simulink model "sim_adc_2nd_1bit_combfilterfix"  (R2022a)
settings: Solver=FixedStepDiscrete  StartTime=0.0  StopTime=Tstop  RelTol=1e-3  EnableMultiTasking=on
values from neighbouring files (symbols this model uses):
  a1 = 0.7752    [Sigmadelta_1bit_CIC.m]
  a2 = 0.215    [Sigmadelta_1bit_CIC.m]
  AMPL = 10^(A_dB/20)    (= 0.501187233627)    [Sigmadelta_1bit_CIC.m]
  c1 = 1    [Sigmadelta_1bit_CIC.m]
  dec = 256    [CIC_scriptexample1.m]    (also in Sigmadelta_1bit_CIC.m = 128)
  ft_sig = tonebin/Bs    [Sigmadelta_1bit_CIC.m]
settings Model: Creator=ceballos  LastModifiedBy=eduyilmet001
settings SolverCC: AlgebraicLoopSolver=TrustRegion
settings DataIOCC: LimitDataPoints=on  SaveFormat=Array  SignalLoggingSaveFormat=ModelDataLogs  ReturnWorkspaceOutputs=off
settings OptimizationCC: BooleanDataType=off  ExpressionDepthLimit=2147483647  LifeSpan=inf
settings DebuggingCC: SaveWithParameterizedLinksMsg=none  UnderspecifiedInitializationDetection=Classic  MergeDetectMultiDrivingBlocksExec=none  SignalResolutionControl=TryResolveAllWithWarning  MultiTaskDSMMsg=warning  MultiTaskCondExecSysMsg=none  FcnCallInpInsideContextMsg=warning  UnconnectedInputMsg=warning  UnconnectedOutputMsg=warning  UnconnectedLineMsg=warning  StateNameClashWarn=warning  SFUnexpectedBacktrackingDiag=warning  SFNoUnconditionalDefaultTransitionDiag=warning  SFExecutionAtInitializationDiag=none  SFMachineParentedDataDiag=warning  ArithmeticOperatorsInVariantConditions=warning
settings HardwareCC: ProdBitPerPointer=32  ProdBitPerSizeT=32  ProdBitPerPtrDiffT=32  ProdLargestAtomicFloat=None  ProdIntDivRoundTo=Undefined  ProdEndianess=Unspecified  ProdWordSize=32  ProdHWDeviceType=32-bit Generic  TargetBitPerPointer=64  TargetBitPerSizeT=64  TargetBitPerPtrDiffT=64  TargetLongLongMode=on  TargetIntDivRoundTo=Zero  TargetEndianess=LittleEndian  TargetWordSize=64  TargetHWDeviceType=MATLAB Host  ProdEqTarget=off
settings ModelReferenceCC: PropagateSignalLabelsOutOfModel=off
settings SFSimCC: SimUseLocalCustomCode=off  CustomCodeUndefinedFunction=UseInterfaceOnly
settings RTWCC: RTWUseLocalCustomCode=off
settings CodeAppCC: StateflowObjectComments=on
settings GRTTargetCC: TargetLangStandard=C89/C90 (ANSI)  CombineOutputUpdateFcns=off  GRTInterface=on
settings ConfigComp: CovMetricSettings=dw  CovSaveCumulativeToWorkspaceVar=on  CovSaveSingleToWorkspaceVar=on  CovExternalEMLEnable=off  CovSFcnEnable=off

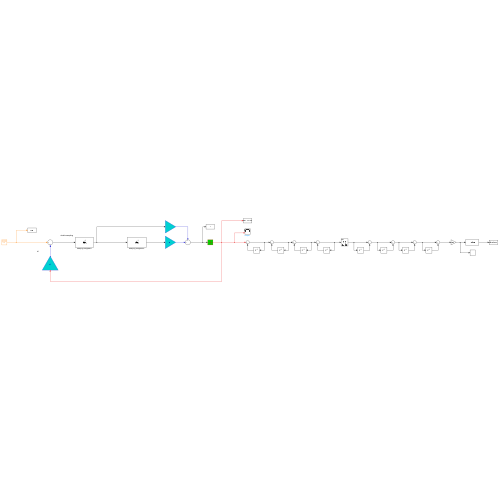
[thumbnail: Simulink's stored preview of the top-level diagram]
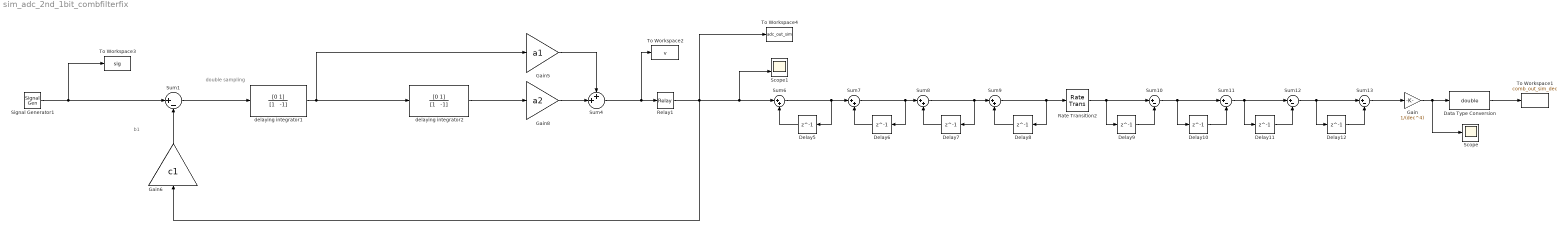
== system sim_adc_2nd_1bit_combfilterfix ==
  note: double sampling
  note: b1
  Data Type Conversion : DataTypeConversion  OutDataTypeStr=double  SaturateOnIntegerOverflow=off  RndMeth=Floor
  Delay{5..12} (8 alike) : Delay  DelayLength=1  InitialCondition=0
  Gain : Gain  Gain=1/(dec^4)
  Gain5 : Gain  Gain=a1  SaturateOnIntegerOverflow=on  OutDataTypeStr=Inherit: Same as input  ParamDataTypeStr=Inherit: Same as input
  Gain6 : Gain  Gain=c1  SaturateOnIntegerOverflow=on  OutDataTypeStr=Inherit: Same as input  ParamDataTypeStr=Inherit: Same as input
  Gain8 : Gain  Gain=a2  SaturateOnIntegerOverflow=on  OutDataTypeStr=Inherit: Same as input  ParamDataTypeStr=Inherit: Same as input
  Rate Transition2 : RateTransition  OutPortSampleTimeOpt=Multiple of input port sample time  OutPortSampleTimeMultiple=dec
  Relay1 : Relay  OffSwitchValue=-eps  OffOutputValue=-1
  Scope : Scope
  Scope1 : Scope  NumInputPorts=2
  Signal Generator1 : SignalGenerator  Amplitude=AMPL  Frequency=ft_sig
  Sum1 : Sum  Inputs=|+-  InputSameDT=on  SaturateOnIntegerOverflow=on  OutDataTypeStr=Inherit: Same as first input
  Sum{10..13} (4 alike) : Sum  Inputs=|+-  AccumDataTypeStr=fixdt(1,32,0)  OutDataTypeStr=Inherit: Same as accumulator
  Sum4 : Sum  Inputs=++|  InputSameDT=on  SaturateOnIntegerOverflow=on  OutDataTypeStr=Inherit: Same as first input
  Sum{6..9} (4 alike) : Sum  Inputs=|++  AccumDataTypeStr=fixdt(1,32,0)  OutDataTypeStr=Inherit: Same as accumulator
  To Workspace1 : ToWorkspace  VariableName=comb_out_sim_dec  SampleTime=-1
  To Workspace2 : ToWorkspace  VariableName=v  SampleTime=1
  To Workspace3 : ToWorkspace  VariableName=sig  SampleTime=1
  To Workspace4 : ToWorkspace  VariableName=adc_out_sim  SampleTime=1
  "delaying integrator1 " : DiscreteFilter  Numerator=[0 1]  Denominator="[1   -1]"  SampleTime=1
  "delaying integrator2 " : DiscreteFilter  Numerator=[0 1]  Denominator="[1   -1]"  SampleTime=1
  wires:
  "delaying integrator1 "/1 -> "delaying integrator2 "/1, Gain5/1
  Sum4/1 -> To Workspace2/1, Relay1/1
  Sum1/1 -> "delaying integrator1 "/1
  "delaying integrator2 "/1 -> Gain8/1
  Gain5/1 -> Sum4/1
  Gain8/1 -> Sum4/2
  Signal Generator1/1 -> Sum1/1, To Workspace3/1
  Gain6/1 -> Sum1/2
  Sum12/1 -> Delay12/1, Sum13/1
  Delay8/1 -> Sum9/2
  Sum11/1 -> Delay11/1, Sum12/1
  Delay11/1 -> Sum12/2
  Sum7/1 -> Sum8/1, Delay6/1
  Sum6/1 -> Sum7/1, Delay5/1
  Delay10/1 -> Sum11/2
  Sum8/1 -> Sum9/1, Delay7/1
  Relay1/1 -> Scope1/2, Sum6/1, Gain6/1, To Workspace4/1
  Rate Transition2/1 -> Delay9/1, Sum10/1
  Sum10/1 -> Delay10/1, Sum11/1
  Delay6/1 -> Sum7/2
  Delay9/1 -> Sum10/2
  Delay12/1 -> Sum13/2
  Sum9/1 -> Rate Transition2/1, Delay8/1
  Delay7/1 -> Sum8/2
  Delay5/1 -> Sum6/2
  Data Type Conversion/1 -> To Workspace1/1
  Sum13/1 -> Gain/1
  Gain/1 -> Scope/1, Data Type Conversion/1
